simulink model "MovingAvg2"  (R2022a)
settings: Solver=FixedStepAuto  StartTime=0.0  StopTime=500  FixedStep=1/360  RelTol=1e-3
undefined symbols (not defined in the file or in its folder): sigbuilder_block
settings Model: Creator=rupak  LastModifiedBy=rupak
settings ConfigComp: DVTestSuiteOptimization=Auto  DVDetectOutOfBounds=on  DVModelReferenceHarness=on  DVHarnessSource=Signal Editor

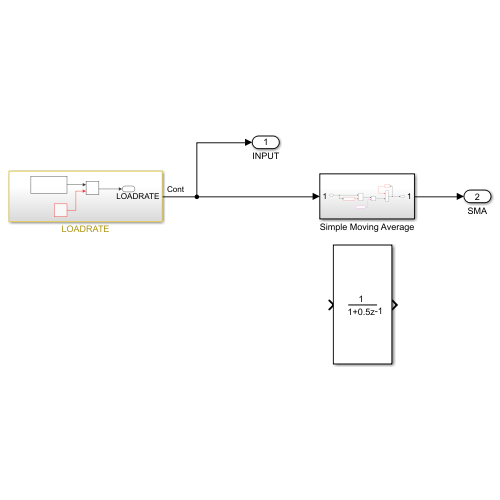
[thumbnail: Simulink's stored preview of the top-level diagram]
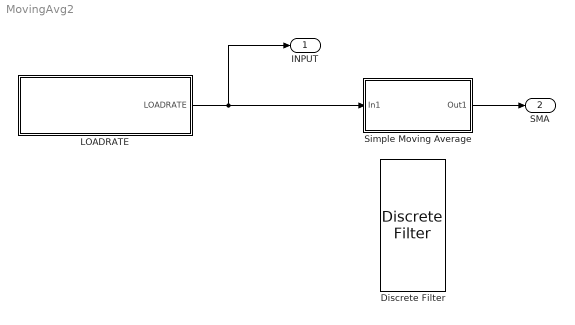
== system MovingAvg2 ==
  Discrete Filter : DiscreteFilter
  LOADRATE : Subsystem
  Simple Moving Average : Subsystem
  INPUT : Outport
  SMA : Outport  Port=2
  wires:
  LOADRATE/1(LOADRATE) -> Simple Moving Average/1(In1), INPUT/1
  Simple Moving Average/1(Out1) -> SMA/1

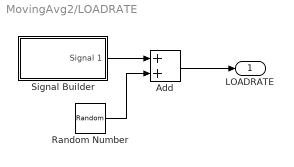
== system MovingAvg2/LOADRATE ==
  Add : Sum
  Random Number : RandomNumber  Mean=5  SampleTime=1/360
  Signal Builder : Subsystem  Tag=STV Subsys  LoadFcn=sigbuilder_block('load');  StartFcn=sigbuilder_block('start');  StopFcn=sigbuilder_block('stop');  ClipboardFcn=sigbuilder_block('clipboard');  mask(Sigbuilder block){tuvar=[0:10]}
      mask help: Simulink:masks:SigbuilderBlock_MD
      mask init:
      | if ~strcmp(get_param(bdroot(gcbh),'SimulationStatus'),'stopped') tuvar = sigbuilder_block('maskInit'); end
      settings: CopyFcn=sigbuilder_block('copy');  DeleteFcn=sigbuilder_block('delete');  ModelCloseFcn=sigbuilder_block('modelClose');  PreSaveFcn=sigbuilder_block('preSave');  PauseFcn=sigbuilder_block('pause');  ContinueFcn=sigbuilder_block('continue');  NameChangeFcn=sigbuilder_block('namechange');  OpenFcn=sigbuilder_block('open',[6 36 1428 675.75 ]);  CloseFcn=sigbuilder_block('close');
      mask Display: plot(0, 0, 100, 100,[2, 2, 32, 32, 2], [68, 8, 8, 68, 68],[32, 2], [38, 38], [32, 19, 2],[53, 60, 44], [32, 17, 17, 2],[16, 16, 31, 31]);txt = getActiveGroup(gcbh);text(2, 100, txt,'verticalAlignment', 'top');
  LOADRATE : Outport
  wires:
  Add/1 -> LOADRATE/1
  Random Number/1 -> Add/2
  Signal Builder/1(Signal 1) -> Add/1

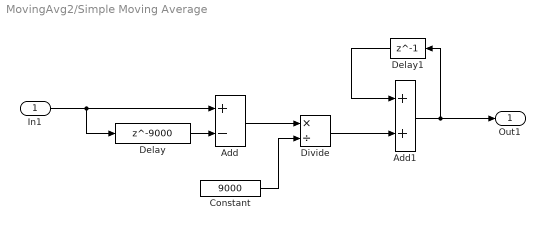
== system MovingAvg2/Simple Moving Average ==
  In1 : Inport
  Add : Sum  Inputs=+-
  Add1 : Sum
  Constant : Constant  Value=9000
  Delay : Delay  DelayLength=9000  InitialCondition=60
  Delay1 : Delay  DelayLength=1  InitialCondition=60
  Divide : Product  Inputs=*/
  Out1 : Outport
  wires:
  Delay/1 -> Add/2
  Delay1/1 -> Add1/1
  Constant/1 -> Divide/2
  In1/1 -> Delay/1, Add/1
  Add/1 -> Divide/1
  Add1/1 -> Out1/1, Delay1/1
  Divide/1 -> Add1/2

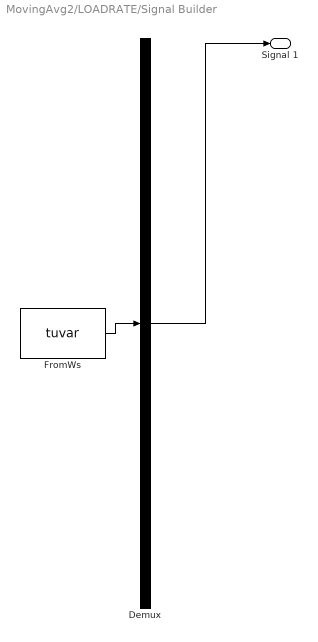
== system MovingAvg2/LOADRATE/Signal Builder ==
  Demux : Demux  Tag=STV Demux  Outputs=1
      settings: DisplayOption=none
  FromWs : FromWorkspace  Tag=STV FromWs  VariableName=tuvar
      SigBuilderData=|
      | common.afterFinalStr = 'Extrapolate'
      | common.sampleTime = 0
      | dataSet.timeRange = [0 500]
      | dataSet.name = 'Group 1'
      | sbobj.Groups.Name = 'Group 1'
      | sbobj.Groups.Signals.Name = 'Signal 1'
      | sbobj.Groups.Signals.XData = [0 5 5 11 13 16 18.5 21 24.5 31 36.5 40 44 50 57 61 61 65 65 71 75 79 81.5 85.5 87.5 89 89.5 93 98 104 108.4 112.5 121.5 133 145 150.5 154.5 157.5 160 162 165.5 170 176.5 181 182.5 184.5 191 199.5 208 217 225.5 231.5 241 250 259.5 266.5 277.5 285 291.5 295.5 299.5 303.5 310.5 315.5 321.5 337.5 346.5 356.5 362 368 374 378.5 385 392.5 399.5 405.5 415 420 424 429.5 433 438 442 446 450 458 465 469.5 475.5 482.5 489.5 500]
      | sbobj.Groups.Signals.YData = [1 95.2 68.2 83 74 55.8 89 73.4 79.8 64.2 90 84.4 66.4 76.4 66 60 47 17.6 30.6 59.6 61.8 47.6 62.4 85.6 77.2 82.2 70 57.4 77.6 35 84.4 56 41 65.6 47 66.6 59.6 72.6 86.4 84.4 55.6 60 33 50.4 73.2 49.8 92 77 59.6 74.6 47.2 57 64.6 48 70 62.8 74.2 53.8 68 64.8 69 53.8 50.8 53.6 37 54.6 47.8 56.2 47 84.8 62.8 66.8 53.6 48.4 62 53.8 75.4 65.4 69 63.8 34.4 63.2 55.8 58 52 65.8 56.6 68 52.4 69 44.4 48]
      | sbobj.Groups.TimeRange = [0 500]
  Signal 1 : Outport  Tag=STV Outport
  wires:
  Demux/1 -> Signal 1/1
  FromWs/1 -> Demux/1
